simulink model "sigma_delta"  (Simulink 7.7)
settings: Solver=FixedStepDiscrete  StartTime=0.0  StopTime=.02  FixedStep=1e-7  RelTol=1e-3
undefined symbols (not defined in the file or in its folder): dfilt, fdesignblkfcn, gcbh
libraries: dsparch4 x1
settings Model: Creator=embed  LastModifiedBy=embed

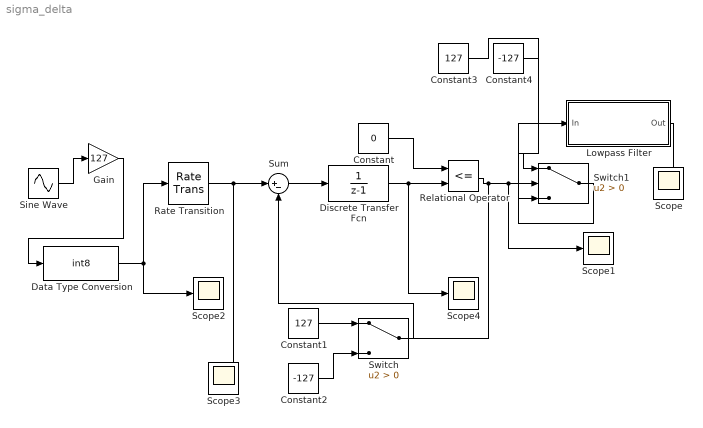
== system sigma_delta ==
  Constant : Constant  Value=0  OutDataTypeStr=fixdt(1,32)
  Constant1 : Constant  Value=127  OutDataTypeStr=fixdt(1,16,7)
  Constant2 : Constant  Value=-127  OutDataTypeStr=fixdt(1,16,7)
  Constant3 : Constant  Value=127  OutDataTypeStr=fixdt(1,16,7)
  Constant4 : Constant  Value=-127  OutDataTypeStr=fixdt(1,16,7)
  Data Type Conversion : DataTypeConversion  OutDataTypeStr=int8
  Discrete Transfer Fcn : DiscreteTransferFcn  Denominator=[1 -1]  SampleTime=-1
  Gain : Gain  Gain=127
  Lowpass Filter : Subsystem  DialogController=fdesignblkfcn  DialogControllerArgs=DataTag1  InitFcn=fdesignblkfcn(gcbh, {'InitFcn'});
      settings: CopyFcn=fdesignblkfcn(gcbh, {'CopyFcn'});
      mask Type: Lowpass Filter
      mask Description: Design a lowpass filter
      mask Help: helpview(mapfilelocation('dsp'), 'dsplowpassfilter');
      mask Display: disp('Lowpass')
  Rate Transition : RateTransition  OutPortSampleTime=1e-7
  Relational Operator : RelationalOperator  Operator=<=  OutDataTypeStr=boolean
  Scope{,1..4} (5 alike) : Scope
      Scope settings: YMin=-150  YMax=150  MaxDataPoints=100000
      Scope2 settings: SaveName=ScopeData2
      Scope3 settings: SaveName=ScopeData3  MaxDataPoints=100000
      Scope4 settings: SaveName=ScopeData4  MaxDataPoints=100000
  Sine Wave : Sin  SineType=Sample based  Samples=195  SampleTime=512/10e6
  Sum : Sum  Inputs=|+-  SampleTime=1e-7
  Switch : Switch  Criteria=u2 > Threshold
  Switch1 : Switch  Criteria=u2 > Threshold
  wires:
  Sum/1 -> Discrete Transfer Fcn/1
  Discrete Transfer Fcn/1 -> Scope4/1, Relational Operator/2
  Relational Operator/1 -> Switch/2, Scope1/1, Switch1/2
  Lowpass Filter/1(Out) -> Scope/1
  Rate Transition/1 -> Scope3/1, Sum/1
  Data Type Conversion/1 -> Rate Transition/1, Scope2/1
  Constant/1 -> Relational Operator/1
  Sine Wave/1 -> Gain/1
  Gain/1 -> Data Type Conversion/1
  Constant1/1 -> Switch/1
  Constant2/1 -> Switch/3
  Switch/1 -> Sum/2
  Switch1/1 -> Lowpass Filter/1(In)
  Constant3/1 -> Switch1/3
  Constant4/1 -> Switch1/1

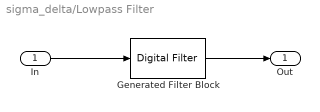
== system sigma_delta/Lowpass Filter ==
  In : Inport
  Generated Filter Block : dsparch4/Digital Filter  Tag=BlockMethodSubSystem  TypePopup=FIR (all zeros)  IIRFiltStruct=Direct form II transposed  AllPoleFiltStruct=Direct form  FIRFiltStruct=Direct form  CoeffSource=Specify via dialog  NumCoeffs=[-0.000946936317809537 -2.72162333860479e-005 -2.6335919972853e-005 -2.47834412951877e-005 -2.22175857538178e-005 -1.89167657788113e-005 -1.45313194653272e-005 -9.33512463243314e-006 -2.98159962757381e-006 4.24981777236742e-006 1.27464371875566e-005 2.21723969268163e-005 3.29691402674294e-005 4.48127936782053e-005 5.80630891369867e-005 7.24420414378393e-005 8.83455063234399e-005 0.000105477197813107 0.000124235906261579 0.00014430357403251 0.000166078415518151 0.000189257145136645 0.000214304479165682 0.000240828710377218 0.000269351989427262 0.000299466891912762 0.00033171193250473 0.000365645435969367 0.000401887987207557 0.000439847267604614 0.000480336237081834 0.000522178967333794 0.000564477964467623 0.000612137553092058 0.000660313988876813 0.000711026975714763 0.000763840681576896 0.000818997540696543 0.000876415589510288 0.00093616641243849 0.000998263033762093 0.0010626916109775 0.00112955992496814 0.00119871702083959 0.00127039896828102 0.00134442385620319 0.00142093243945678 0.00149977824046326 0.00158114053474192 0.00166484319752406 0.00175106640233611 0.00183959383183368 0.0019305865376695 0.00202383338562877 0.00211953540246256 0.00221740267441258 0.00231768198489104 0.00242005595049001 0.0025247780560344 0.00263152464890196 0.00274060513044316 0.00285162133846843 0.00296499916287444 0.00307996002490556 0.00319648787314148 0.00331556157574858 0.00343601620254624 0.00355827669744225 0.00368212141925327 0.00380751517338386 0.00393437887384302 0.0040626042074764 0.00419213223636467 0.00432282198983211 0.0044546740421762 0.00458738677039578 0.00472113867121641 0.00485559521979596 0.0049907984847287 0.00512647485659833 0.00526269397947842 0.00539917714369395 0.00553599456947779 0.0056728404686921 0.00580975605962333 0.00594645403779541 0.00608299408340746 0.00621903753622254 0.00635468311659099 0.00648956083226777 0.00662377065351528 0.00675695079819393 0.0068892494938503 0.00702028084761598 0.00715029623637521 0.00727862982030324 0.00740534826497956 0.00753061562394503 0.00765395064091215 0.00777538195527508 0.00789475422091703 0.0080119196901898 0.00812679665312778 0.00823922417804936 0.00834910580780309 0.00845631137421039 0.00856078716334677 0.00866219439080728 0.00876076772409298 0.00885612492696164 0.00894833397080948 0.0090370998587087 0.00912251625901015 0.00920431254485797 0.0092825953836171 0.00935708684776009 0.00942786971162687 0.00949470390229565 0.0095576800636104 0.00961654276190778 0.00967142659224662 0.00972205151409875 0.00976855445679685 0.00981067306360764 0.00984858787500796 0.0098820486004043 0.00991133821564246 0.00993599716722742 0.00995622572280445 0.00997203921923607 0.00998332481509755 0.00999009693637216 0.00999237078524871 0.00999009693637216 0.00998332481509755 0.00997203921923607 0.00995622572280445 0.00993599716722742 0.00991133821564246 0.0098820486004043 0.00984858787500796 0.00981067306360764 0.00976855445679685 0.00972205151409875 0.00967142659224662 0.00961654276190778 0.0095576800636104 0.00949470390229565 0.00942786971162687 0.00935708684776009 0.0092825953836171 0.00920431254485797 0.00912251625901015 0.0090370998587087 0.00894833397080948 0.00885612492696164 0.00876076772409298 0.00866219439080728 0.00856078716334677 0.00845631137421039 0.00834910580780309 0.00823922417804936 0.00812679665312778 0.0080119196901898 0.00789475422091703 0.00777538195527508 0.00765395064091215 0.00753061562394503 0.00740534826497956 0.00727862982030324 0.00715029623637521 0.00702028084761598 0.0068892494938503 0.00675695079819393 0.00662377065351528 0.00648956083226777 0.00635468311659099 0.00621903753622254 0.00608299408340746 0.00594645403779541 0.00580975605962333 0.0056728404686921 0.00553599456947779 0.00539917714369395 0.00526269397947842 0.00512647485659833 0.0049907984847287 0.00485559521979596 0.00472113867121641 0.00458738677039578 0.0044546740421762 0.00432282198983211 0.00419213223636467 0.0040626042074764 0.00393437887384302 0.00380751517338386 0.00368212141925327 0.00355827669744225 ...(+1399 chars)]  DenCoeffs=[1 0.1]  BiQuadCoeffs=[1 0.3 0.4 1 0.1 0.2]  LatticeCoeffs=[0.2 0.4]  denIgnore=on  FiltPerSampPopup=One filter per frame  IC=0  ICnum=0  ICden=0  roundingMode=Floor  overflowMode=off  ScaleValues=1  scaleValueFracLength=14  stageInFracLength=15  stageOutFracLength=15  FilterSource=Specify via dialog  dfiltObjectName=dfilt.dffir([1 2 1])  InputProcessing=Columns as channels (frame based)
  Out : Outport
  wires:
  In/1 -> Generated Filter Block/1
  Generated Filter Block/1 -> Out/1
